simulink model "L4_sim2"  (R2024b)
settings: Solver=VariableStepAuto  StartTime=0.0  StopTime=100  RelTol=1e-3
values from neighbouring files (symbols this model uses):
  I = diag([Ix, Iy, Iz])    [Task1.m]    (also in Task3.m)
  q_0 = [0 0 0 1]'    [Task3.m]
  w_0 = [0.45, 0.52, 0.55]'    [Task1.m]    (also in Task3.m = [0.3, 0.15, 0.6]')
libraries: matrix_library x1, vrlib x1
settings Model: Creator=alejandromunozvazquez  LastModifiedBy=alejandromunozvazquez

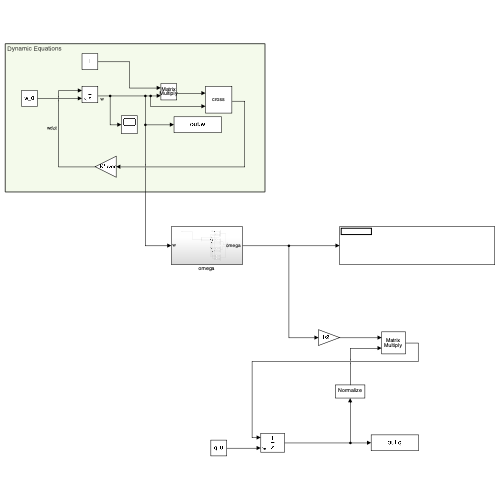
[thumbnail: Simulink's stored preview of the top-level diagram]
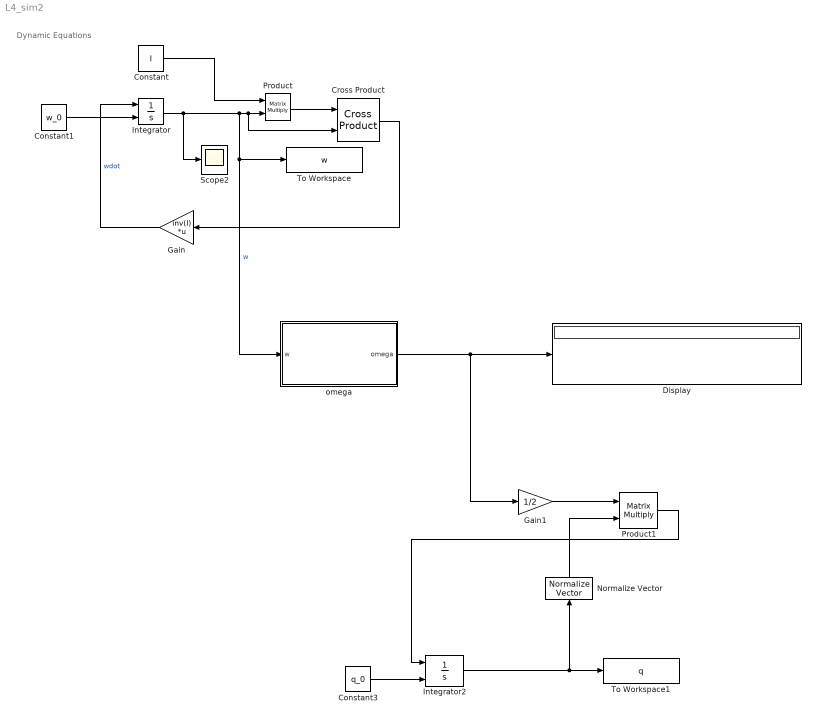
== system L4_sim2 ==
  note: Dynamic Equations
  Constant : Constant  Value=I
  Constant1 : Constant  Value=w_0
  Constant3 : Constant  Value=q_0
  Cross Product : matrix_library/Cross Product
  Display : Display
  Gain : Gain  Gain=inv(I)  Multiplication=Matrix(K*u) (u vector)
  Gain1 : Gain  Gain=1/2
  Integrator : Integrator  InitialConditionSource=external
  Integrator2 : Integrator  InitialConditionSource=external
  Normalize Vector : vrlib/Utilities/Normalize Vector  maxzero=0
  Product : Product  Multiplication=Matrix(*)
  Product1 : Product  Multiplication=Matrix(*)
  Scope2 : Scope
  To Workspace : ToWorkspace  VariableName=w  SampleTime=-1
  To Workspace1 : ToWorkspace  VariableName=q  SampleTime=-1
  "omega " : Subsystem
  wires:
  Gain/1 -> Integrator/1  "wdot"
  Integrator/1 -> Scope2/1, Product/2, Cross Product/2, "omega "/1(w), To Workspace/1  "w"
  Constant/1 -> Product/1
  Product/1 -> Cross Product/1
  Cross Product/1 -> Gain/1
  Constant1/1 -> Integrator/2
  Product1/1 -> Integrator2/1
  Constant3/1 -> Integrator2/2
  Gain1/1 -> Product1/1
  Integrator2/1 -> Normalize Vector/1, To Workspace1/1
  "omega "/1(omega) -> Gain1/1, Display/1
  Normalize Vector/1 -> Product1/2

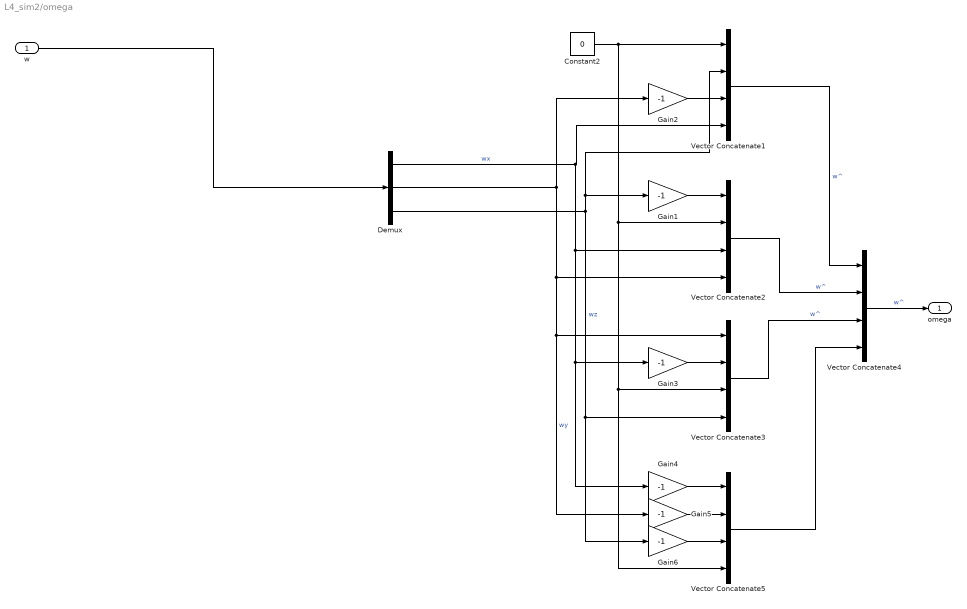
== system L4_sim2/omega  ==
  w : Inport
  Constant2 : Constant  Value=0
  Demux : Demux  Outputs=3
  Gain{1..6} (6 alike) : Gain  Gain=-1
  Vector Concatenate{1..3,5} (4 alike) : Concatenate  NumInputs=4  Mode=Multidimensional array
  Vector Concatenate4 : Concatenate  NumInputs=4  Mode=Multidimensional array  ConcatenateDimension=2
  omega : Outport
  wires:
  w/1 -> Demux/1
  Vector Concatenate4/1 -> omega/1  "w^"
  Demux/2 -> Gain5/1, Vector Concatenate3/1, Vector Concatenate2/4, Gain2/1  "wy"
  Vector Concatenate1/1 -> Vector Concatenate4/1  "w^"
  Demux/1 -> Gain4/1, Gain3/1, Vector Concatenate2/3, Vector Concatenate1/4  "wx"
  Vector Concatenate3/1 -> Vector Concatenate4/3  "w^"
  Vector Concatenate2/1 -> Vector Concatenate4/2  "w^"
  Demux/3 -> Gain6/1, Vector Concatenate3/4, Gain1/1, Vector Concatenate1/2  "wz"
  Vector Concatenate5/1 -> Vector Concatenate4/4
  Gain2/1 -> Vector Concatenate1/3
  Gain1/1 -> Vector Concatenate2/1
  Gain3/1 -> Vector Concatenate3/2
  Constant2/1 -> Vector Concatenate5/4, Vector Concatenate3/3, Vector Concatenate2/2, Vector Concatenate1/1
  Gain4/1 -> Vector Concatenate5/1
  Gain6/1 -> Vector Concatenate5/3
  Gain5/1 -> Vector Concatenate5/2
